simulink model "DCmotor"  (R2025b)
settings: Solver=VariableStepAuto  StartTime=0.0  StopTime=10.0  RelTol=1e-3
undefined symbols (not defined in the file): b, J, K, L, R
settings Model: Creator=lando  LastModifiedBy=lando

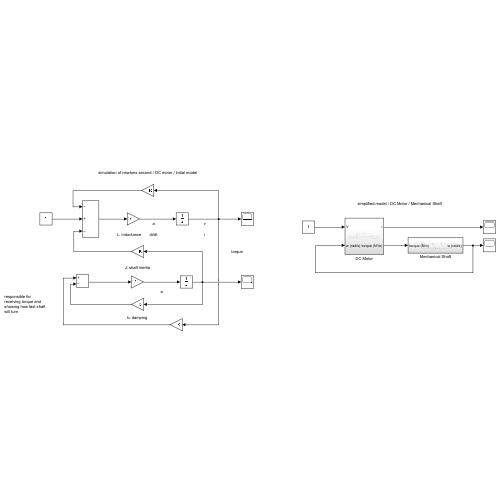
[thumbnail: Simulink's stored preview of the top-level diagram]
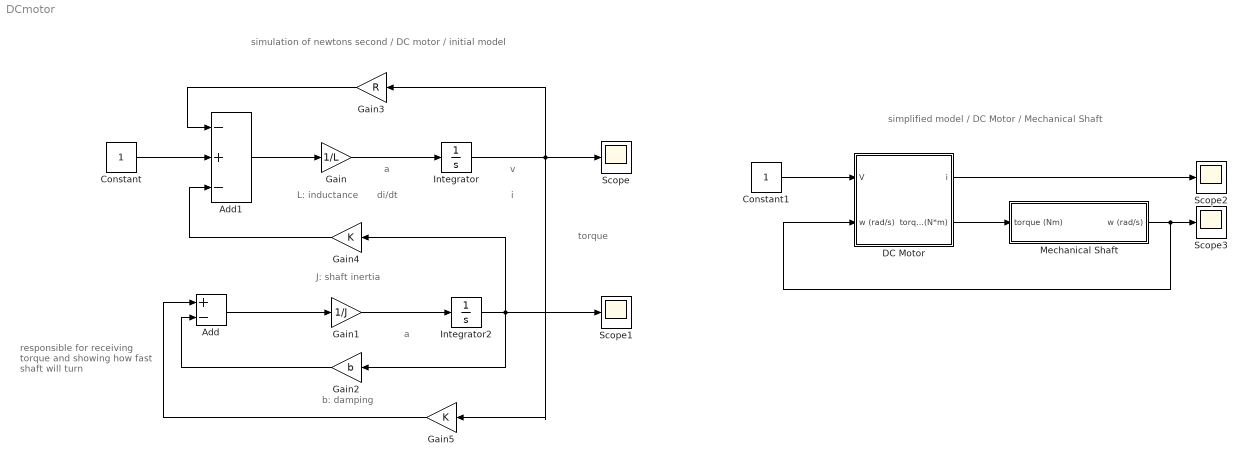
== system DCmotor ==
  note: simplified model / DC Motor / Mechanical Shaft
  note: responsible for receiving torque and showing how fast shaft will turn
  note: torque
  note: i
  note: di/dt
  note: L: inductance
  note: J: shaft inertia
  note: b: damping
  note: simulation of newtons second / DC motor / initial model
  note: v
  note: a
  note: a
  Add : Sum  Inputs=+-
  Add1 : Sum  Inputs=-+-
  Constant : Constant
  Constant1 : Constant
  DC Motor : Subsystem
  Gain : Gain  Gain=1/L
  Gain1 : Gain  Gain=1/J
  Gain2 : Gain  Gain=b
  Gain3 : Gain  Gain=R
  Gain4 : Gain  Gain=K
  Gain5 : Gain  Gain=K
  Integrator : Integrator
  Integrator2 : Integrator
  Mechanical Shaft : Subsystem
  Scope{,1..3} (4 alike) : Scope
      Scope settings: ActiveDisplayYMinimum=-27.364364744610466  ActiveDisplayYMaximum=28.354887063422446
      Scope1 settings: ActiveDisplayYMinimum=-23.475567549399003  ActiveDisplayYMaximum=27.063436358113847
      Scope2 settings: ActiveDisplayYMinimum=-3.4489804569392613  ActiveDisplayYMaximum=3.062445658996392  DataLoggingVariableName=ScopeData2
      Scope3 settings: ActiveDisplayYMinimum=-23.475567549399003  ActiveDisplayYMaximum=27.063436358113847  DataLoggingVariableName=ScopeData3
  wires:
  Integrator/1 -> Gain5/1, Gain3/1, Scope/1
  Gain/1 -> Integrator/1
  Gain1/1 -> Integrator2/1
  Add/1 -> Gain1/1
  Integrator2/1 -> Gain4/1, Scope1/1, Gain2/1
  Gain2/1 -> Add/2
  Add1/1 -> Gain/1
  Constant/1 -> Add1/2
  Gain3/1 -> Add1/1
  Gain4/1 -> Add1/3
  Gain5/1 -> Add/1
  Mechanical Shaft/1(w (rad/s)) -> DC Motor/2(w (rad/s)), Scope3/1
  Constant1/1 -> DC Motor/1(V)
  DC Motor/1(i) -> Scope2/1
  DC Motor/2(torque (N*m)) -> Mechanical Shaft/1(torque (Nm))

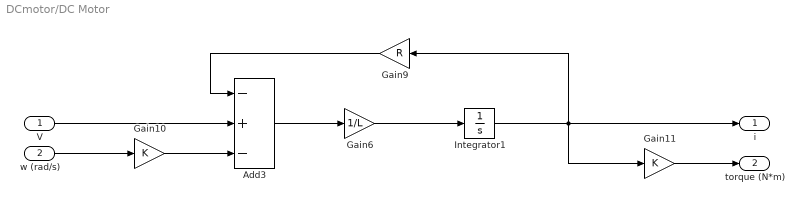
== system DCmotor/DC Motor ==
  V : Inport
  w (rad/s) : Inport  Port=2
  Add3 : Sum  Inputs=-+-
  Gain10 : Gain  Gain=K
  Gain11 : Gain  Gain=K
  Gain6 : Gain  Gain=1/L
  Gain9 : Gain  Gain=R
  Integrator1 : Integrator
  i : Outport
  torque (N*m) : Outport  Port=2
  wires:
  Gain11/1 -> torque (N*m)/1
  Integrator1/1 -> i/1, Gain9/1, Gain11/1
  w (rad/s)/1 -> Gain10/1
  Gain10/1 -> Add3/3
  Gain9/1 -> Add3/1
  Gain6/1 -> Integrator1/1
  Add3/1 -> Gain6/1
  V/1 -> Add3/2

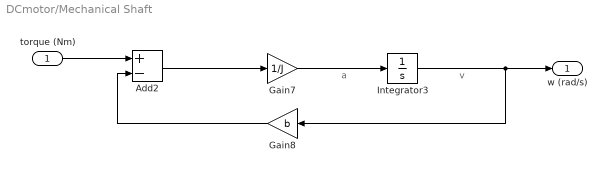
== system DCmotor/Mechanical Shaft ==
  note: v
  note: a
  torque (Nm) : Inport
  Add2 : Sum  Inputs=+-
  Gain7 : Gain  Gain=1/J
  Gain8 : Gain  Gain=b
  Integrator3 : Integrator
  w (rad/s) : Outport
  wires:
  Gain8/1 -> Add2/2
  Add2/1 -> Gain7/1
  Integrator3/1 -> Gain8/1, w (rad/s)/1
  Gain7/1 -> Integrator3/1
  torque (Nm)/1 -> Add2/1
